simulink model "mpc_optimalcost"  (R2023a)
settings: Solver=ode5  StartTime=0  StopTime=Tstop  RelTol=1e-3
values from neighbouring files (symbols this model uses):
  Ts = 0.2    [mpcoptimalcost1.m]
  x0 = [0;0;0]    [mpcoptimalcost1.m]
undefined symbols (not defined in the file or in its folder): A, B, C, D
libraries: mpclib x2
settings Model: ExtModeTrigMode=oneshot  Creator=The MathWorks, Inc.  LastModifiedBy=The MathWorks, Inc.
settings SolverCC: AlgebraicLoopSolver=TrustRegion  MaxZcPerStep=1
settings DataIOCC: SaveFormat=Array  ReturnWorkspaceOutputs=off  SignalLoggingName=sigsOut
settings OptimizationCC: BooleanDataType=off  ExpressionDepthLimit=2147483647  InitFltsAndDblsToZero=on  LifeSpan=inf
settings DebuggingCC: SaveWithParameterizedLinksMsg=none  UnderspecifiedInitializationDetection=Classic  MergeDetectMultiDrivingBlocksExec=none  CheckExecutionContextPreStartOutputMsg=on  SignalResolutionControl=TryResolveAllWithWarning  MultiTaskDSMMsg=warning  MultiTaskCondExecSysMsg=none  IntegerOverflowMsg=none  FcnCallInpInsideContextMsg=warning  UnconnectedInputMsg=warning  UnconnectedOutputMsg=warning  UnconnectedLineMsg=warning  StateNameClashWarn=warning  SFUnexpectedBacktrackingDiag=warning  SFNoUnconditionalDefaultTransitionDiag=warning  SFExecutionAtInitializationDiag=none  IntegerSaturationMsg=none  ArithmeticOperatorsInVariantConditions=warning
settings HardwareCC: ProdBitPerPointer=32  ProdBitPerSizeT=32  ProdBitPerPtrDiffT=32  ProdLargestAtomicFloat=None  ProdIntDivRoundTo=Undefined  ProdEndianess=Unspecified  ProdWordSize=32  ProdHWDeviceType=32-bit Generic  TargetUnknown=on
settings ModelReferenceCC: EnableRefExpFcnMdlSchedulingChecks=on  PropagateSignalLabelsOutOfModel=off
settings SFSimCC: SimUseLocalCustomCode=off  CustomCodeUndefinedFunction=UseInterfaceOnly
settings RTWCC: RTWUseLocalCustomCode=off  DLArmComputeVersion=19.05
settings CodeAppCC: StateflowObjectComments=on
settings GRTTargetCC: TargetFcnLib=ansi_tfl_tmw.mat  TargetLangStandard=C89/C90 (ANSI)  CombineOutputUpdateFcns=off  GRTInterface=on
settings ConfigComp: CovMetricSettings=dw  CovSaveCumulativeToWorkspaceVar=on  CovSaveSingleToWorkspaceVar=on  CovExternalEMLEnable=off  CovSFcnEnable=off

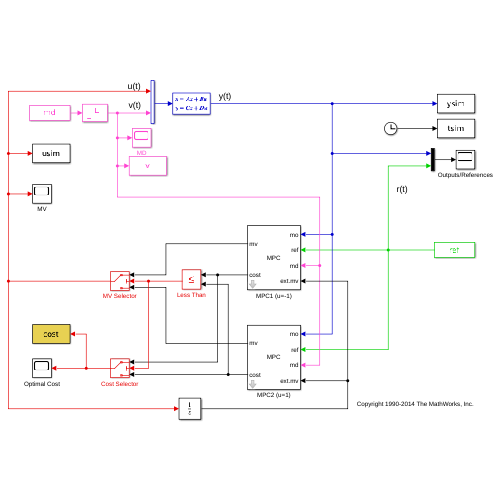
[thumbnail: Simulink's stored preview of the top-level diagram]
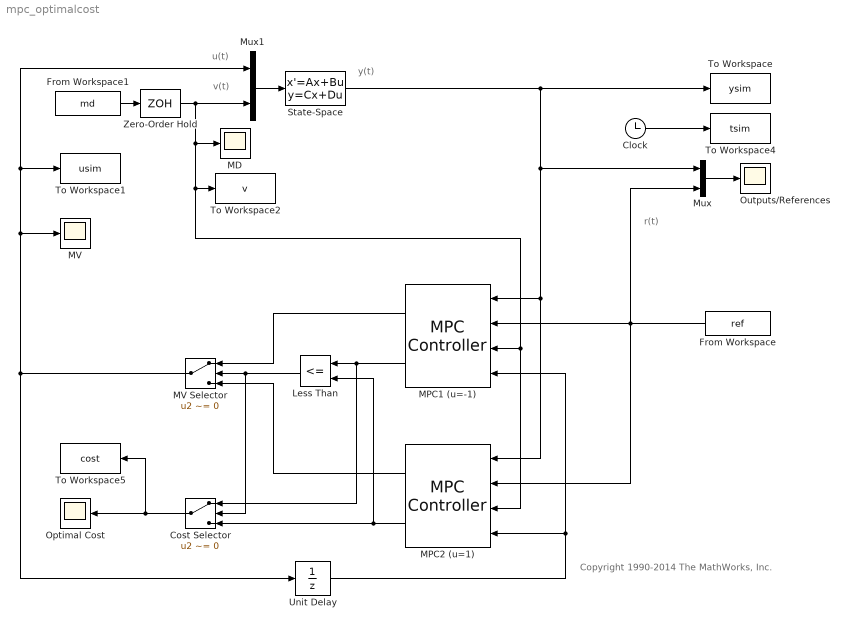
== system mpc_optimalcost ==
  note: u(t)
  note: y(t)
  note: r(t)
  note: v(t)
  note: Copyright 1990-2014 The MathWorks, Inc.
  Clock : Clock
  Cost Selector : Switch  Criteria=u2 ~= 0  SaturateOnIntegerOverflow=off  InputSameDT=off
  From Workspace : FromWorkspace  VariableName=ref  ZeroCross=off  OutputAfterFinalValue=Holding final value
  From Workspace1 : FromWorkspace  VariableName=md  ZeroCross=off  OutputAfterFinalValue=Holding final value
  Less Than : RelationalOperator  Operator=<=  OutDataTypeStr=boolean  InputSameDT=off
  MD : Scope
  MPC1 (u=-1) : mpclib/MPC Controller  mpcobj=mpc1  x0=[]  is_multiple=0  enable_value=0  return_u0=off  updateMPCinCallerWorkspace=on  md_inport=on  mv_inport=on  uref_inport=off  return_cost=on  return_mvseq=off  return_qpstatus=off  return_xseq=off  return_state=off  return_ovseq=off  state_inport=off  umin_inport=off  umax_inport=off  ymin_inport=off  ymax_inport=off  cc_inport=off  ywt_inport=off  uwt_inport=off  duwt_inport=off  rhoeps_inport=off  pm_inport=off  MaximumP=10  HorizonChoice=FixedHorizon  n_ts=0.2  n_p=20  n_mv=1  n_md=1  n_ud=0  n_mo=1  n_uo=0  BlockDataType=double  SampleTimeInherited=off  switch_inport=off
  MPC2 (u=1) : mpclib/MPC Controller  mpcobj=mpc2  x0=[]  is_multiple=0  enable_value=0  return_u0=off  updateMPCinCallerWorkspace=on  md_inport=on  mv_inport=on  uref_inport=off  return_cost=on  return_mvseq=off  return_qpstatus=off  return_xseq=off  return_state=off  return_ovseq=off  state_inport=off  umin_inport=off  umax_inport=off  ymin_inport=off  ymax_inport=off  cc_inport=off  ywt_inport=off  uwt_inport=off  duwt_inport=off  rhoeps_inport=off  pm_inport=off  MaximumP=10  HorizonChoice=FixedHorizon  n_ts=0.2  n_p=20  n_mv=1  n_md=1  n_ud=0  n_mo=1  n_uo=0  BlockDataType=double  SampleTimeInherited=off  switch_inport=off
  MV : Scope
  MV Selector : Switch  Criteria=u2 ~= 0  SaturateOnIntegerOverflow=off  InputSameDT=off
  Mux : Mux  Inputs=2
  Mux1 : Mux  Inputs=2
  Optimal Cost : Scope
  Outputs/References : Scope
  State-Space : StateSpace  A=A  B=B  C=C  D=D  InitialCondition=x0
  To Workspace : ToWorkspace  VariableName=ysim  SampleTime=-1
      settings: MaxDataPoints=Inf
  To Workspace1 : ToWorkspace  VariableName=usim  SampleTime=-1
      settings: MaxDataPoints=Inf
  To Workspace2 : ToWorkspace  VariableName=v  SampleTime=-1
      settings: MaxDataPoints=Inf
  To Workspace4 : ToWorkspace  VariableName=tsim  SampleTime=-1
      settings: MaxDataPoints=Inf
  To Workspace5 : ToWorkspace  VariableName=cost  SampleTime=-1
      settings: MaxDataPoints=Inf
  Unit Delay : UnitDelay  SampleTime=-1  HasFrameUpgradeWarning=on
  Zero-Order Hold : ZeroOrderHold  SampleTime=Ts
  wires:
  Mux1/1 -> State-Space/1
  Mux/1 -> Outputs/References/1
  From Workspace/1 -> Mux/2, MPC1 (u=-1)/2, MPC2 (u=1)/2
  Clock/1 -> To Workspace4/1
  State-Space/1 -> Mux/1, MPC1 (u=-1)/1, MPC2 (u=1)/1, To Workspace/1
  From Workspace1/1 -> Zero-Order Hold/1
  Zero-Order Hold/1 -> Mux1/2, MD/1, To Workspace2/1, MPC1 (u=-1)/3, MPC2 (u=1)/3
  MPC1 (u=-1)/1 -> MV Selector/1
  MPC1 (u=-1)/2 -> Less Than/1, Cost Selector/1
  MPC2 (u=1)/2 -> Cost Selector/3, Less Than/2
  MV Selector/1 -> Unit Delay/1, Mux1/1, To Workspace1/1, MV/1
  MPC2 (u=1)/1 -> MV Selector/3
  Less Than/1 -> MV Selector/2, Cost Selector/2
  Cost Selector/1 -> To Workspace5/1, Optimal Cost/1
  Unit Delay/1 -> MPC2 (u=1)/4, MPC1 (u=-1)/4
